simulink model "MPC_regulator"  (R2021a)
settings: Solver=VariableStepAuto  StartTime=0.0  StopTime=10.0  RelTol=1e-3
settings Model: Creator=chshx  LastModifiedBy=apple

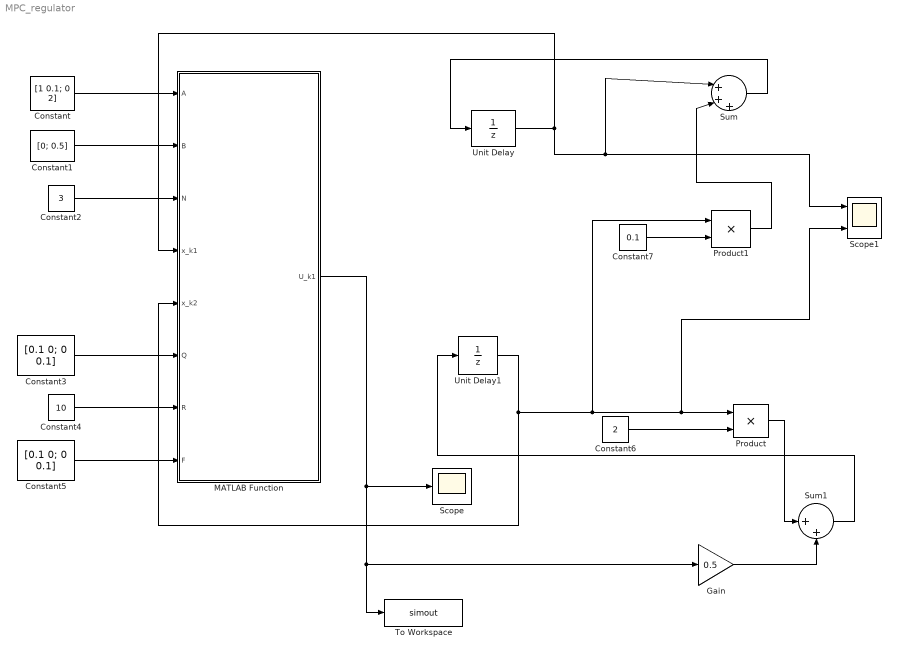
== system MPC_regulator ==
  Constant : Constant  Value=[1 0.1; 0 2]  VectorParams1D=off
  Constant1 : Constant  Value=[0; 0.5]  VectorParams1D=off
  Constant2 : Constant  Value=3
  Constant3 : Constant  Value=[0.1 0; 0 0.1]  VectorParams1D=off
  Constant4 : Constant  Value=10
  Constant5 : Constant  Value=[0.1 0; 0 0.1]  VectorParams1D=off
  Constant6 : Constant  Value=2
  Constant7 : Constant  Value=0.1
  Gain : Gain  Gain=0.5
  MATLAB Function : MATLAB Function  TreatAsAtomicUnit=on
  Product : Product
  Product1 : Product
  Scope : Scope
  Scope1 : Scope  NumInputPorts=2
  Sum : Sum  Inputs=|+++
  Sum1 : Sum  Inputs=|++
  To Workspace : ToWorkspace  VariableName=simout  SampleTime=-1
  Unit Delay : UnitDelay  SampleTime=-1  HasFrameUpgradeWarning=on
  Unit Delay1 : UnitDelay  SampleTime=-1  HasFrameUpgradeWarning=on
  wires:
  Constant/1 -> MATLAB Function/1(A)
  Constant1/1 -> MATLAB Function/2(B)
  Constant2/1 -> MATLAB Function/3(N)
  Constant3/1 -> MATLAB Function/6(Q)
  Constant4/1 -> MATLAB Function/7(R)
  Constant5/1 -> MATLAB Function/8(F)
  MATLAB Function/1(U_k1) -> To Workspace/1, Gain/1, Scope/1
  Constant6/1 -> Product/2
  Gain/1 -> Sum1/2
  Product/1 -> Sum1/1
  Sum1/1 -> Unit Delay1/1
  Unit Delay1/1 -> Product1/1, Scope1/2, Product/1, MATLAB Function/5(x_k2)
  Constant7/1 -> Product1/2
  Product1/1 -> Sum/2
  Unit Delay/1 -> Sum/1, Scope1/1, MATLAB Function/4(x_k1)
  Sum/1 -> Unit Delay/1

== matlab function MPC_regulator/MATLAB Function ==
  data: A input; U_k1 output; B input; N input; x_k1 input; x_k2 input; Q input; R input; F input
function U_k1  = MPC_Zero_Ref(A, B, N, x_k1, x_k2, Q, R, F)
%UNTITLED 此处提供此函数的摘要
%   此处提供详细说明
coder.extrinsic('quadprog');
n = size(A, 1); 
p = size(B, 2);
M= [eye(n); zeros(N*n, n)];
C = zeros((N+1)*n, N*p);
x_k = [x_k1 x_k2]';
U_k1 = 10;

tmp = eye(n);
for i = 1 : N
    rows = i * n + (1 : n);
    C(rows, :) = [tmp*B, C(rows-n, 1 : end-p)];
    tmp = A * tmp;
    M(rows, :) = tmp;
end

S_q = size(Q, 1);
S_r = size(R, 1);

Q_bar = zeros((N+1)*S_q, (N+1)*S_q);
for i = 0 : N-1
    Q_bar(i*S_q+1 : (i+1)*S_q, i*S_q+1 :(i+1)*S_q) = Q;
end
Q_bar(N*S_q+1 : (N+1)*S_q, N*S_q+1 :(N+1)*S_q) = F;

R_bar = zeros(N*S_r, N*S_r);
for i = 0 : N-1
    R_bar(i*S_r+1 : (i+1)*S_r, i*S_r+1 : (i+1)*S_r) = R;
end

G = M' * Q_bar * M;
E = C' * Q_bar * M;
H = C' * Q_bar * C + R_bar;

f = (x_k' * E')';
U_K = quadprog(H, f);
U_k1 = U_K(1);
